simulink model "model_mamdani_25_square_charge"  (R2014b)
settings: Solver=ode45  StartTime=0.0  StopTime=1000  RelTol=1e-3
libraries: fuzblock x1
settings Model: Creator=João  LastModifiedBy=Joaquim
settings SolverCC: ZeroCrossControl=DisableAll  ZeroCrossAlgorithm=Adaptive

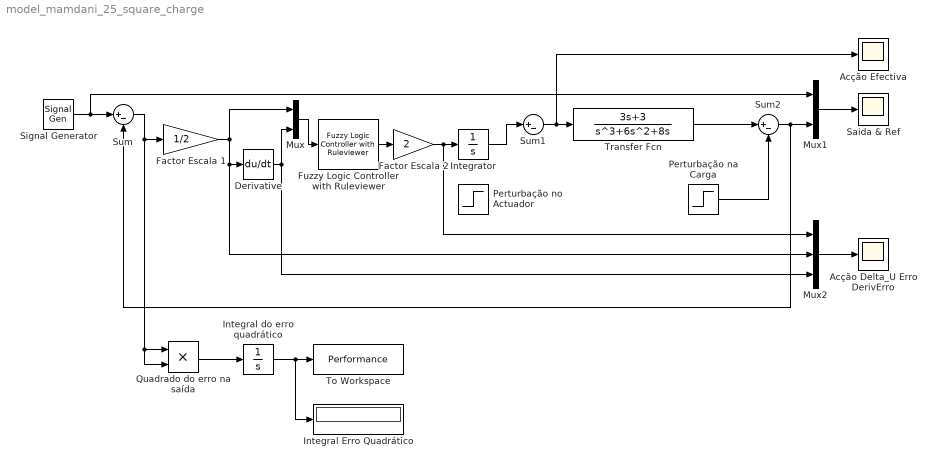
== system model_mamdani_25_square_charge ==
  Acção Delta_U Erro DerivErro : Scope
  Acção Efectiva : Scope
      settings: SaveName=ScopeData2
  Derivative : Derivative
  Factor Escala 1 : Gain  Gain=1/2
  Factor Escala 2 : Gain  Gain=2
  Fuzzy Logic Controller with Ruleviewer : fuzblock/Fuzzy Logic  Controller  with Ruleviewer  fismatrix=mamdani_25  Ts=1
  Integral Erro Quadrático : Display
  Integral do erro quadrático : Integrator
  Integrator : Integrator
  Mux : Mux  Inputs=2
  Mux1 : Mux  Inputs=2
  Mux2 : Mux  Inputs=3
  Perturbação na Carga : Step  SampleTime=0
  Perturbação no Actuador : Step  SampleTime=0
  Quadrado do erro na saída : Product
  Saida & Ref : Scope
      settings: MaxDataPoints=50000
  Signal Generator : SignalGenerator  WaveForm=square  Amplitude=-1  Frequency=0.01  Units=rad/sec
  Sum : Sum  Inputs=|+-
  Sum1 : Sum  Inputs=|+-
  Sum2 : Sum  Inputs=|+-
  To Workspace : ToWorkspace  VariableName=Performance  SaveFormat=Timeseries  SampleTime=-1
  Transfer Fcn : TransferFcn  Numerator=[3 3]  Denominator=[1 6 8 0]
  wires:
  Signal Generator/1 -> Mux1/1, Sum/1
  Sum/1 -> Quadrado do erro na saída/2, Quadrado do erro na saída/1, Factor Escala 1/1
  Derivative/1 -> Mux2/3, Mux/2
  Factor Escala 1/1 -> Mux/1, Mux2/2, Derivative/1
  Factor Escala 2/1 -> Mux2/1, Integrator/1
  Integrator/1 -> Sum1/1
  Sum1/1 -> Acção Efectiva/1, Transfer Fcn/1
  Transfer Fcn/1 -> Sum2/1
  Sum2/1 -> Sum/2, Mux1/2
  Mux1/1 -> Saida & Ref/1
  Mux2/1 -> Acção Delta_U Erro DerivErro/1
  Quadrado do erro na saída/1 -> Integral do erro quadrático/1
  Integral do erro quadrático/1 -> Integral Erro Quadrático/1, To Workspace/1
  Fuzzy Logic Controller with Ruleviewer/1 -> Factor Escala 2/1
  Mux/1 -> Fuzzy Logic Controller with Ruleviewer/1
  Perturbação na Carga/1 -> Sum2/2
